simulink model "s_function_test"  (R2024b)
settings: Solver=FixedStepAuto  StartTime=0.0  StopTime=10.0  RelTol=1e-3
settings Model: Creator=agaydos  LastModifiedBy=agaydos

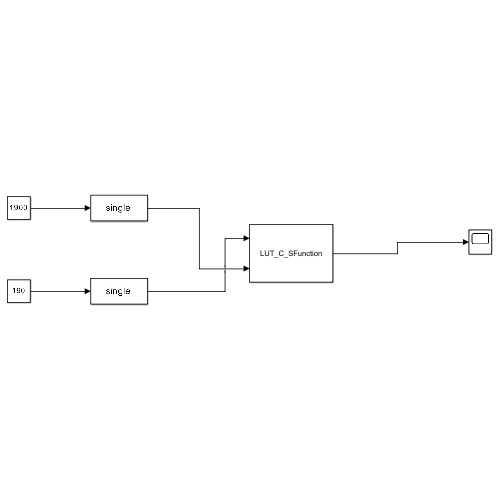
[thumbnail: Simulink's stored preview of the top-level diagram]
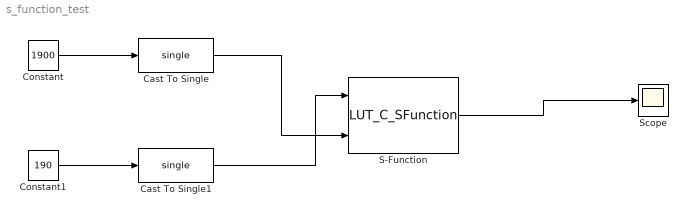
== system s_function_test ==
  Cast To Single : DataTypeConversion  OutDataTypeStr=single  SaturateOnIntegerOverflow=off  RndMeth=Floor
  Cast To Single1 : DataTypeConversion  OutDataTypeStr=single  SaturateOnIntegerOverflow=off  RndMeth=Floor
  Constant : Constant  Value=1900
  Constant1 : Constant  Value=190
  S-Function : S-Function  FunctionName=LUT_C_SFunction  SFunctionDeploymentMode=off  EnableBusSupport=off
  Scope : Scope
  wires:
  S-Function/1 -> Scope/1
  Constant/1 -> Cast To Single/1
  Constant1/1 -> Cast To Single1/1
  Cast To Single/1 -> S-Function/2
  Cast To Single1/1 -> S-Function/1
